simulink model "sm_vehicle_2axle_heave_roll_mu"  (R2025b)
settings: Solver=ode23t  StartTime=0.0  StopTime=14.2  MaxStep=0.2  RelTol=1e-3  AbsTol=1e-3  EnableMultiTasking=on
PostLoadFcn:
  | sm_vehicle_2axle_heave_roll_param
  | sm_vehicle_2axle_heave_roll_scene
  | sm_vehicle_2axle_heave_roll_config_maneuver(bdroot,VehicleData,'plateau');
  | set_param([bdroot '/Vehicle'],'popup_surface_conditions','Checker Right');
StartFcn:
  | tic
StopFcn:
  | Elapsed_Sim_Time = toc;
undefined symbols (not defined in the file): brake_trqTs, Disc, FL, FR, Hydraulic, InitVehicle, Mode, RL, RR, SceneData, valve_maxA, valve_maxO, VehicleData, X, Y, Z
libraries: fl_lib x92, sm_lib x43, nesl_utility x40, sm_vehicle_utilities_lib x21, sdlc_lib x8, SimscapeFluids_lib x8, simulink x2, simulink_extras x1
(part 5 of 5)

== system sm_vehicle_2axle_heave_roll_mu/Brakes/Brakes/Disc/Actuator/Hydraulic/Return Spring FR ==
  Damper : fl_lib/Mechanical/Translational Elements/Translational Damper  D=D N/(m/s)  v_specify=off  v_priority=None  v=0 m/s  v_nominal_specify=off  v_nominal_value=1  v_nominal_unit=m/s  f_specify=off  f_priority=None  f=0 N  f_nominal_specify=off  f_nominal_value=1  f_nominal_unit=N
  Spring : fl_lib/Mechanical/Translational Elements/Translational Spring  spr_rate=spr_rate N/m  v_specify=off  v_priority=None  v=0 m/s  v_nominal_specify=off  v_nominal_value=1  v_nominal_unit=m/s  f_specify=off  f_priority=None  f=0 N  f_nominal_specify=off  f_nominal_value=1  f_nominal_unit=N  x_specify=off  x_priority=High  x=0 m  x_nominal_specify=off  x_nominal_value=1  x_nominal_unit=m
  R : PMIOPort  Side=Right
  C : PMIOPort  Port=2  Side=Left
  connections:
  Damper/LConn1 -- R/RConn1 -- Spring/LConn1
  C/RConn1 -- Damper/RConn1 -- Spring/RConn1

== system sm_vehicle_2axle_heave_roll_mu/Brakes/Brakes/Disc/Actuator/Hydraulic/Return Spring RL ==
  Damper : fl_lib/Mechanical/Translational Elements/Translational Damper  D=D N/(m/s)  v_specify=off  v_priority=None  v=0 m/s  v_nominal_specify=off  v_nominal_value=1  v_nominal_unit=m/s  f_specify=off  f_priority=None  f=0 N  f_nominal_specify=off  f_nominal_value=1  f_nominal_unit=N
  Spring : fl_lib/Mechanical/Translational Elements/Translational Spring  spr_rate=spr_rate N/m  v_specify=off  v_priority=None  v=0 m/s  v_nominal_specify=off  v_nominal_value=1  v_nominal_unit=m/s  f_specify=off  f_priority=None  f=0 N  f_nominal_specify=off  f_nominal_value=1  f_nominal_unit=N  x_specify=off  x_priority=High  x=0 m  x_nominal_specify=off  x_nominal_value=1  x_nominal_unit=m
  R : PMIOPort  Side=Right
  C : PMIOPort  Port=2  Side=Left
  connections:
  R/RConn1 -- Damper/LConn1 -- Spring/LConn1
  C/RConn1 -- Spring/RConn1 -- Damper/RConn1

== system sm_vehicle_2axle_heave_roll_mu/Brakes/Brakes/Disc/Actuator/Hydraulic/Return Spring RR ==
  Damper : fl_lib/Mechanical/Translational Elements/Translational Damper  D=D N/(m/s)  v_specify=off  v_priority=None  v=0 m/s  v_nominal_specify=off  v_nominal_value=1  v_nominal_unit=m/s  f_specify=off  f_priority=None  f=0 N  f_nominal_specify=off  f_nominal_value=1  f_nominal_unit=N
  Spring : fl_lib/Mechanical/Translational Elements/Translational Spring  spr_rate=spr_rate N/m  v_specify=off  v_priority=None  v=0 m/s  v_nominal_specify=off  v_nominal_value=1  v_nominal_unit=m/s  f_specify=off  f_priority=None  f=0 N  f_nominal_specify=off  f_nominal_value=1  f_nominal_unit=N  x_specify=off  x_priority=High  x=0 m  x_nominal_specify=off  x_nominal_value=1  x_nominal_unit=m
  R : PMIOPort  Side=Right
  C : PMIOPort  Port=2  Side=Left
  connections:
  Spring/RConn1 -- Damper/RConn1 -- C/RConn1
  Spring/LConn1 -- R/RConn1 -- Damper/LConn1

== system sm_vehicle_2axle_heave_roll_mu/Brakes/Brakes/Disc/Actuator/Ideal/Actuator Dynamics FL ==
  In : Inport
  Gain : Gain  Gain=1./b
  Integrator : Integrator  InitialCondition=x_initial.*b
  Sum : Sum  Inputs=|+-  InputSameDT=on  SaturateOnIntegerOverflow=on  OutDataTypeStr=Inherit: Same as first input
  Out : Outport  VectorParamsAs1DForOutWhenUnconnected=off
  wires:
  Sum/1 -> Integrator/1
  In/1 -> Sum/1
  Integrator/1 -> Gain/1
  Gain/1 -> Sum/2, Out/1

== system sm_vehicle_2axle_heave_roll_mu/Brakes/Brakes/Disc/Actuator/Ideal/Actuator Dynamics FR ==
  In : Inport
  Gain : Gain  Gain=1./b
  Integrator : Integrator  InitialCondition=x_initial.*b
  Sum : Sum  Inputs=|+-  InputSameDT=on  SaturateOnIntegerOverflow=on  OutDataTypeStr=Inherit: Same as first input
  Out : Outport  VectorParamsAs1DForOutWhenUnconnected=off
  wires:
  Gain/1 -> Out/1, Sum/2
  Integrator/1 -> Gain/1
  In/1 -> Sum/1
  Sum/1 -> Integrator/1

== system sm_vehicle_2axle_heave_roll_mu/Brakes/Brakes/Disc/Actuator/Ideal/Actuator Dynamics RL ==
  In : Inport
  Gain : Gain  Gain=1./b
  Integrator : Integrator  InitialCondition=x_initial.*b
  Sum : Sum  Inputs=|+-  InputSameDT=on  SaturateOnIntegerOverflow=on  OutDataTypeStr=Inherit: Same as first input
  Out : Outport  VectorParamsAs1DForOutWhenUnconnected=off
  wires:
  Gain/1 -> Out/1, Sum/2
  Integrator/1 -> Gain/1
  In/1 -> Sum/1
  Sum/1 -> Integrator/1

== system sm_vehicle_2axle_heave_roll_mu/Brakes/Brakes/Disc/Actuator/Ideal/Actuator Dynamics RR ==
  In : Inport
  Gain : Gain  Gain=1./b
  Integrator : Integrator  InitialCondition=x_initial.*b
  Sum : Sum  Inputs=|+-  InputSameDT=on  SaturateOnIntegerOverflow=on  OutDataTypeStr=Inherit: Same as first input
  Out : Outport  VectorParamsAs1DForOutWhenUnconnected=off
  wires:
  Sum/1 -> Integrator/1
  In/1 -> Sum/1
  Integrator/1 -> Gain/1
  Gain/1 -> Sum/2, Out/1

== system sm_vehicle_2axle_heave_roll_mu/Brakes/Brakes/Disc/Actuator/Ideal/Front Piston Area ==
  Cylinder Bore : Constant  Value=d_caliper_bore_f
  Gain pi div 4 : Gain  Gain=pi/4
  Square : Math  Operator=square  SignedPower=on
  area : Outport  VectorParamsAs1DForOutWhenUnconnected=off
  wires:
  Square/1 -> Gain pi div 4/1
  Cylinder Bore/1 -> Square/1
  Gain pi div 4/1 -> area/1

== system sm_vehicle_2axle_heave_roll_mu/Brakes/Brakes/Disc/Actuator/Ideal/Rear Piston Area ==
  Cylinder Bore : Constant  Value=d_caliper_bore_r
  Gain pi div 4 : Gain  Gain=pi/4
  Square : Math  Operator=square  SignedPower=on
  area : Outport  VectorParamsAs1DForOutWhenUnconnected=off
  wires:
  Gain pi div 4/1 -> area/1
  Cylinder Bore/1 -> Square/1
  Square/1 -> Gain pi div 4/1

== system sm_vehicle_2axle_heave_roll_mu/Brakes/Brakes/Disc/Actuator/Ideal/Return Spring FL ==
  Damper : fl_lib/Mechanical/Translational Elements/Translational Damper  D=D N/(m/s)  v_specify=off  v_priority=None  v=0 m/s  v_nominal_specify=off  v_nominal_value=1  v_nominal_unit=m/s  f_specify=off  f_priority=None  f=0 N  f_nominal_specify=off  f_nominal_value=1  f_nominal_unit=N
  Spring : fl_lib/Mechanical/Translational Elements/Translational Spring  spr_rate=spr_rate N/m  v_specify=off  v_priority=None  v=0 m/s  v_nominal_specify=off  v_nominal_value=1  v_nominal_unit=m/s  f_specify=off  f_priority=None  f=0 N  f_nominal_specify=off  f_nominal_value=1  f_nominal_unit=N  x_specify=off  x_priority=High  x=0 m  x_nominal_specify=off  x_nominal_value=1  x_nominal_unit=m
  R : PMIOPort  Side=Right
  C : PMIOPort  Port=2  Side=Left
  connections:
  Damper/LConn1 -- R/RConn1 -- Spring/LConn1
  C/RConn1 -- Damper/RConn1 -- Spring/RConn1

== system sm_vehicle_2axle_heave_roll_mu/Brakes/Brakes/Disc/Actuator/Ideal/Return Spring FR ==
  Damper : fl_lib/Mechanical/Translational Elements/Translational Damper  D=D N/(m/s)  v_specify=off  v_priority=None  v=0 m/s  v_nominal_specify=off  v_nominal_value=1  v_nominal_unit=m/s  f_specify=off  f_priority=None  f=0 N  f_nominal_specify=off  f_nominal_value=1  f_nominal_unit=N
  Spring : fl_lib/Mechanical/Translational Elements/Translational Spring  spr_rate=spr_rate N/m  v_specify=off  v_priority=None  v=0 m/s  v_nominal_specify=off  v_nominal_value=1  v_nominal_unit=m/s  f_specify=off  f_priority=None  f=0 N  f_nominal_specify=off  f_nominal_value=1  f_nominal_unit=N  x_specify=off  x_priority=High  x=0 m  x_nominal_specify=off  x_nominal_value=1  x_nominal_unit=m
  R : PMIOPort  Side=Right
  C : PMIOPort  Port=2  Side=Left
  connections:
  Spring/RConn1 -- Damper/RConn1 -- C/RConn1
  Spring/LConn1 -- R/RConn1 -- Damper/LConn1

== system sm_vehicle_2axle_heave_roll_mu/Brakes/Brakes/Disc/Actuator/Ideal/Return Spring RL ==
  Damper : fl_lib/Mechanical/Translational Elements/Translational Damper  D=D N/(m/s)  v_specify=off  v_priority=None  v=0 m/s  v_nominal_specify=off  v_nominal_value=1  v_nominal_unit=m/s  f_specify=off  f_priority=None  f=0 N  f_nominal_specify=off  f_nominal_value=1  f_nominal_unit=N
  Spring : fl_lib/Mechanical/Translational Elements/Translational Spring  spr_rate=spr_rate N/m  v_specify=off  v_priority=None  v=0 m/s  v_nominal_specify=off  v_nominal_value=1  v_nominal_unit=m/s  f_specify=off  f_priority=None  f=0 N  f_nominal_specify=off  f_nominal_value=1  f_nominal_unit=N  x_specify=off  x_priority=High  x=0 m  x_nominal_specify=off  x_nominal_value=1  x_nominal_unit=m
  R : PMIOPort  Side=Right
  C : PMIOPort  Port=2  Side=Left
  connections:
  Damper/RConn1 -- Spring/RConn1 -- C/RConn1
  Spring/LConn1 -- Damper/LConn1 -- R/RConn1

== system sm_vehicle_2axle_heave_roll_mu/Brakes/Brakes/Disc/Actuator/Ideal/Return Spring RR ==
  Damper : fl_lib/Mechanical/Translational Elements/Translational Damper  D=D N/(m/s)  v_specify=off  v_priority=None  v=0 m/s  v_nominal_specify=off  v_nominal_value=1  v_nominal_unit=m/s  f_specify=off  f_priority=None  f=0 N  f_nominal_specify=off  f_nominal_value=1  f_nominal_unit=N
  Spring : fl_lib/Mechanical/Translational Elements/Translational Spring  spr_rate=spr_rate N/m  v_specify=off  v_priority=None  v=0 m/s  v_nominal_specify=off  v_nominal_value=1  v_nominal_unit=m/s  f_specify=off  f_priority=None  f=0 N  f_nominal_specify=off  f_nominal_value=1  f_nominal_unit=N  x_specify=off  x_priority=High  x=0 m  x_nominal_specify=off  x_nominal_value=1  x_nominal_unit=m
  R : PMIOPort  Side=Right
  C : PMIOPort  Port=2  Side=Left
  connections:
  Damper/LConn1 -- R/RConn1 -- Spring/LConn1
  C/RConn1 -- Damper/RConn1 -- Spring/RConn1

== system sm_vehicle_2axle_heave_roll_mu/Brakes/Brakes/Disc/Actuator/Valves/Return Spring FL ==
  Damper : fl_lib/Mechanical/Translational Elements/Translational Damper  D=D N/(m/s)  v_specify=off  v_priority=None  v=0 m/s  v_nominal_specify=off  v_nominal_value=1  v_nominal_unit=m/s  f_specify=off  f_priority=None  f=0 N  f_nominal_specify=off  f_nominal_value=1  f_nominal_unit=N
  Spring : fl_lib/Mechanical/Translational Elements/Translational Spring  spr_rate=spr_rate N/m  v_specify=off  v_priority=None  v=0 m/s  v_nominal_specify=off  v_nominal_value=1  v_nominal_unit=m/s  f_specify=off  f_priority=None  f=0 N  f_nominal_specify=off  f_nominal_value=1  f_nominal_unit=N  x_specify=off  x_priority=High  x=0 m  x_nominal_specify=off  x_nominal_value=1  x_nominal_unit=m
  R : PMIOPort  Side=Right
  C : PMIOPort  Port=2  Side=Left
  connections:
  Damper/LConn1 -- R/RConn1 -- Spring/LConn1
  C/RConn1 -- Damper/RConn1 -- Spring/RConn1

== system sm_vehicle_2axle_heave_roll_mu/Brakes/Brakes/Disc/Actuator/Valves/Return Spring FR ==
  Damper : fl_lib/Mechanical/Translational Elements/Translational Damper  D=D N/(m/s)  v_specify=off  v_priority=None  v=0 m/s  v_nominal_specify=off  v_nominal_value=1  v_nominal_unit=m/s  f_specify=off  f_priority=None  f=0 N  f_nominal_specify=off  f_nominal_value=1  f_nominal_unit=N
  Spring : fl_lib/Mechanical/Translational Elements/Translational Spring  spr_rate=spr_rate N/m  v_specify=off  v_priority=None  v=0 m/s  v_nominal_specify=off  v_nominal_value=1  v_nominal_unit=m/s  f_specify=off  f_priority=None  f=0 N  f_nominal_specify=off  f_nominal_value=1  f_nominal_unit=N  x_specify=off  x_priority=High  x=0 m  x_nominal_specify=off  x_nominal_value=1  x_nominal_unit=m
  R : PMIOPort  Side=Right
  C : PMIOPort  Port=2  Side=Left
  connections:
  Spring/RConn1 -- Damper/RConn1 -- C/RConn1
  Spring/LConn1 -- R/RConn1 -- Damper/LConn1

== system sm_vehicle_2axle_heave_roll_mu/Brakes/Brakes/Disc/Actuator/Valves/Return Spring RL ==
  Damper : fl_lib/Mechanical/Translational Elements/Translational Damper  D=D N/(m/s)  v_specify=off  v_priority=None  v=0 m/s  v_nominal_specify=off  v_nominal_value=1  v_nominal_unit=m/s  f_specify=off  f_priority=None  f=0 N  f_nominal_specify=off  f_nominal_value=1  f_nominal_unit=N
  Spring : fl_lib/Mechanical/Translational Elements/Translational Spring  spr_rate=spr_rate N/m  v_specify=off  v_priority=None  v=0 m/s  v_nominal_specify=off  v_nominal_value=1  v_nominal_unit=m/s  f_specify=off  f_priority=None  f=0 N  f_nominal_specify=off  f_nominal_value=1  f_nominal_unit=N  x_specify=off  x_priority=High  x=0 m  x_nominal_specify=off  x_nominal_value=1  x_nominal_unit=m
  R : PMIOPort  Side=Right
  C : PMIOPort  Port=2  Side=Left
  connections:
  Damper/RConn1 -- Spring/RConn1 -- C/RConn1
  Spring/LConn1 -- Damper/LConn1 -- R/RConn1

== system sm_vehicle_2axle_heave_roll_mu/Brakes/Brakes/Disc/Actuator/Valves/Return Spring RR ==
  Damper : fl_lib/Mechanical/Translational Elements/Translational Damper  D=D N/(m/s)  v_specify=off  v_priority=None  v=0 m/s  v_nominal_specify=off  v_nominal_value=1  v_nominal_unit=m/s  f_specify=off  f_priority=None  f=0 N  f_nominal_specify=off  f_nominal_value=1  f_nominal_unit=N
  Spring : fl_lib/Mechanical/Translational Elements/Translational Spring  spr_rate=spr_rate N/m  v_specify=off  v_priority=None  v=0 m/s  v_nominal_specify=off  v_nominal_value=1  v_nominal_unit=m/s  f_specify=off  f_priority=None  f=0 N  f_nominal_specify=off  f_nominal_value=1  f_nominal_unit=N  x_specify=off  x_priority=High  x=0 m  x_nominal_specify=off  x_nominal_value=1  x_nominal_unit=m
  R : PMIOPort  Side=Right
  C : PMIOPort  Port=2  Side=Left
  connections:
  Damper/LConn1 -- R/RConn1 -- Spring/LConn1
  C/RConn1 -- Damper/RConn1 -- Spring/RConn1

== system sm_vehicle_2axle_heave_roll_mu/Brakes/Brakes/Disc/Actuator/Valves/Sensing pFL ==
  Hydraulic Pressure Sensor : fl_lib/Isothermal Liquid/Sensors/Pressure Sensor (IL)  pressure_measure=foundation.enum.pressure_measure.difference
      settings: InternalSimscapePortConfiguration="{\"Bottom\":[],\"Left\":[{\"id\":\"A\",\"label\":\"A\",\"type\":\"foundation.isothermal_liquid.isothermal_liquid\"}],\"Right\":[{\"id\":\"B\",\"label\":\"B\",\"type\":\"foundation.isothermal_liquid.isothermal_liquid\"},{\"id\":\"P\",\"label\":\"P\",\"type\":\"output\"}],\"Top\":[]}"
      settings: LibrarySourceBlock=|
      | fl_lib/Hydraulic/Hydraulic Sensors/Hydraulic Pressure
      | Sensor
  Hydraulic Reference : fl_lib/Isothermal Liquid/Elements/Reservoir (IL)  reservoir_type=foundation.enum.constant_controlled.constant  pressure_spec=foundation.enum.pressure_spec.atmospheric  reservoir_pressure=0.101325 MPa
      settings: LibrarySourceBlock=fl_lib/Hydraulic/Hydraulic Elements/Hydraulic Reference
  PS-Simulink Converter : nesl_utility/PS-Simulink Converter  PhysicalDomain=network_engine_domain  SubClassName=ps_output  LeftPortType=input  RightPortType=output  PseudoPeriodic=off  Frequencies=[]  VectorFormat=1-D array  Unit=psi  AffineConversion=off
  A : PMIOPort  Side=Left
  p : Outport  VectorParamsAs1DForOutWhenUnconnected=off
  wires:
  PS-Simulink Converter/1 -> p/1
  connections:
  Hydraulic Pressure Sensor/RConn2 -- PS-Simulink Converter/LConn1
  Hydraulic Pressure Sensor/LConn1 -- A/RConn1
  Hydraulic Reference/LConn1 -- Hydraulic Pressure Sensor/RConn1

== system sm_vehicle_2axle_heave_roll_mu/Brakes/Brakes/Disc/Actuator/Valves/Sensing pFR ==
  Hydraulic Pressure Sensor : fl_lib/Isothermal Liquid/Sensors/Pressure Sensor (IL)  pressure_measure=foundation.enum.pressure_measure.difference
      settings: InternalSimscapePortConfiguration="{\"Bottom\":[],\"Left\":[{\"id\":\"A\",\"label\":\"A\",\"type\":\"foundation.isothermal_liquid.isothermal_liquid\"}],\"Right\":[{\"id\":\"B\",\"label\":\"B\",\"type\":\"foundation.isothermal_liquid.isothermal_liquid\"},{\"id\":\"P\",\"label\":\"P\",\"type\":\"output\"}],\"Top\":[]}"
      settings: LibrarySourceBlock=|
      | fl_lib/Hydraulic/Hydraulic Sensors/Hydraulic Pressure
      | Sensor
  Hydraulic Reference : fl_lib/Isothermal Liquid/Elements/Reservoir (IL)  reservoir_type=foundation.enum.constant_controlled.constant  pressure_spec=foundation.enum.pressure_spec.atmospheric  reservoir_pressure=0.101325 MPa
      settings: LibrarySourceBlock=fl_lib/Hydraulic/Hydraulic Elements/Hydraulic Reference
  PS-Simulink Converter : nesl_utility/PS-Simulink Converter  PhysicalDomain=network_engine_domain  SubClassName=ps_output  LeftPortType=input  RightPortType=output  PseudoPeriodic=off  Frequencies=[]  VectorFormat=1-D array  Unit=psi  AffineConversion=off
  A : PMIOPort  Side=Left
  p : Outport  VectorParamsAs1DForOutWhenUnconnected=off
  wires:
  PS-Simulink Converter/1 -> p/1
  connections:
  Hydraulic Reference/LConn1 -- Hydraulic Pressure Sensor/RConn1
  Hydraulic Pressure Sensor/LConn1 -- A/RConn1
  Hydraulic Pressure Sensor/RConn2 -- PS-Simulink Converter/LConn1

== system sm_vehicle_2axle_heave_roll_mu/Brakes/Brakes/Disc/Actuator/Valves/Sensing pRL ==
  Hydraulic Pressure Sensor : fl_lib/Isothermal Liquid/Sensors/Pressure Sensor (IL)  pressure_measure=foundation.enum.pressure_measure.difference
      settings: InternalSimscapePortConfiguration="{\"Bottom\":[],\"Left\":[{\"id\":\"A\",\"label\":\"A\",\"type\":\"foundation.isothermal_liquid.isothermal_liquid\"}],\"Right\":[{\"id\":\"B\",\"label\":\"B\",\"type\":\"foundation.isothermal_liquid.isothermal_liquid\"},{\"id\":\"P\",\"label\":\"P\",\"type\":\"output\"}],\"Top\":[]}"
      settings: LibrarySourceBlock=|
      | fl_lib/Hydraulic/Hydraulic Sensors/Hydraulic Pressure
      | Sensor
  Hydraulic Reference : fl_lib/Isothermal Liquid/Elements/Reservoir (IL)  reservoir_type=foundation.enum.constant_controlled.constant  pressure_spec=foundation.enum.pressure_spec.atmospheric  reservoir_pressure=0.101325 MPa
      settings: LibrarySourceBlock=fl_lib/Hydraulic/Hydraulic Elements/Hydraulic Reference
  PS-Simulink Converter : nesl_utility/PS-Simulink Converter  PhysicalDomain=network_engine_domain  SubClassName=ps_output  LeftPortType=input  RightPortType=output  PseudoPeriodic=off  Frequencies=[]  VectorFormat=1-D array  Unit=psi  AffineConversion=off
  A : PMIOPort  Side=Left
  p : Outport  VectorParamsAs1DForOutWhenUnconnected=off
  wires:
  PS-Simulink Converter/1 -> p/1
  connections:
  Hydraulic Reference/LConn1 -- Hydraulic Pressure Sensor/RConn1
  Hydraulic Pressure Sensor/LConn1 -- A/RConn1
  Hydraulic Pressure Sensor/RConn2 -- PS-Simulink Converter/LConn1

== system sm_vehicle_2axle_heave_roll_mu/Brakes/Brakes/Disc/Actuator/Valves/Sensing pRR ==
  Hydraulic Pressure Sensor : fl_lib/Isothermal Liquid/Sensors/Pressure Sensor (IL)  pressure_measure=foundation.enum.pressure_measure.difference
      settings: InternalSimscapePortConfiguration="{\"Bottom\":[],\"Left\":[{\"id\":\"A\",\"label\":\"A\",\"type\":\"foundation.isothermal_liquid.isothermal_liquid\"}],\"Right\":[{\"id\":\"B\",\"label\":\"B\",\"type\":\"foundation.isothermal_liquid.isothermal_liquid\"},{\"id\":\"P\",\"label\":\"P\",\"type\":\"output\"}],\"Top\":[]}"
      settings: LibrarySourceBlock=|
      | fl_lib/Hydraulic/Hydraulic Sensors/Hydraulic Pressure
      | Sensor
  Hydraulic Reference : fl_lib/Isothermal Liquid/Elements/Reservoir (IL)  reservoir_type=foundation.enum.constant_controlled.constant  pressure_spec=foundation.enum.pressure_spec.atmospheric  reservoir_pressure=0.101325 MPa
      settings: LibrarySourceBlock=fl_lib/Hydraulic/Hydraulic Elements/Hydraulic Reference
  PS-Simulink Converter : nesl_utility/PS-Simulink Converter  PhysicalDomain=network_engine_domain  SubClassName=ps_output  LeftPortType=input  RightPortType=output  PseudoPeriodic=off  Frequencies=[]  VectorFormat=1-D array  Unit=psi  AffineConversion=off
  A : PMIOPort  Side=Left
  p : Outport  VectorParamsAs1DForOutWhenUnconnected=off
  wires:
  PS-Simulink Converter/1 -> p/1
  connections:
  Hydraulic Pressure Sensor/RConn2 -- PS-Simulink Converter/LConn1
  Hydraulic Pressure Sensor/LConn1 -- A/RConn1
  Hydraulic Reference/LConn1 -- Hydraulic Pressure Sensor/RConn1

== system sm_vehicle_2axle_heave_roll_mu/Brakes/Brakes/Disc/Actuator/Valves/Valves FL ==
  S : Inport
  Actuator Dynamics : Subsystem  mask(First-order lag supporting vector signals){b=brkTs, x_initial=0}
      mask prompts: b "Filter time constant"; x_initial "Initial output"
      mask help: Models a lag of the form 1/(b*s+1) where s is the Laplace operator.
  Demux : Demux  Outputs=2
  Orifice Apply : SimscapeFluids_lib/Isothermal Liquid/Valves & Orifices/Orifices/Orifice (IL)  orifice_type=foundation.enum.constant_variable.variable  constant_orifice_spec=fluids.isothermal_liquid.valves_orifices.orifices.enum.constant_orifice_spec.area  variable_orifice_spec=1  orifice_area_constant=1e-3 m^2  p_diff_TLU_constant=[-4, -3, -2, -1, -.5, 0, .5, 1, 2, 3, 4] MPa  vol_flow_TLU_constant=[-2.44, -2.12, -1.68, -1.22, -.84, 0, .85, 1.21, 1.7, 2.09, 2.41] .* 1e-3 m^3/s  S_min=(open_max_apply)/(area_max_apply)*(1e-12) - (0) m  del_S=(-(0) + (open_max_apply)) - ((open_max_apply)/(area_max_apply)*(1e-12) - (0)) m  open_orientation=1  area_max=area_max_apply m^2  area_leak=1e-12 m^2  S_TLU=[-.002, 0, .002, .005, .015] - (0) m  orifice_area_TLU=[1e-09, 2.0352e-07, 4.0736e-05, .00011438, .00034356] m^2  area=inf m^2  Cd=0.7  Re_c=150  smoothing_factor=0  pressure_recovery=false  S_vol_flow_TLU=[-.002, 0, .002, .005, .015] - (0) m  p_diff_TLU=[-10000000, -5000000, -2000000, 2000000, 5000000, 10000000] Pa  vol_flow_TLU=[-1e-07, -7.0711e-08, -4.4721e-08, 4.4721e-08, 7.0711e-08, 1e-07; -2.0352e-05, -1.4391e-05, -9.1017e-06, 9.1017e-06, 1.4391e-05, 2.0352e-05; -.0040736, -.0028805, -.0018218, .0018218, .0028805, .0040736; -.011438, -.0080879, -.0051152, .0051152, .0080879, .011438; -.034356, -.024293, -.015364, .015364, .024293, .034356] m^3/s
      settings: LibrarySourceBlock=sh_lib/Orifices/Variable Orifice  InternalSimscapePortConfiguration="{\"Bottom\":[],\"Left\":[{\"id\":\"A\",\"label\":\"A\",\"type\":\"foundation.isothermal_liquid.isothermal_liquid\"},{\"id\":\"S\",\"label\":\"S\",\"type\":\"input\"}],\"Right\":[{\"id\":\"B\",\"label\":\"B\",\"type\":\"foundation.isothermal_liquid.isothermal_liquid\"}],\"Top\":[]}"
  Orifice Release : SimscapeFluids_lib/Isothermal Liquid/Valves & Orifices/Orifices/Orifice (IL)  orifice_type=foundation.enum.constant_variable.variable  constant_orifice_spec=fluids.isothermal_liquid.valves_orifices.orifices.enum.constant_orifice_spec.area  variable_orifice_spec=1  orifice_area_constant=1e-3 m^2  p_diff_TLU_constant=[-4, -3, -2, -1, -.5, 0, .5, 1, 2, 3, 4] MPa  vol_flow_TLU_constant=[-2.44, -2.12, -1.68, -1.22, -.84, 0, .85, 1.21, 1.7, 2.09, 2.41] .* 1e-3 m^3/s  S_min=(open_max_rel)/(area_max_rel)*(1e-12) - (0) m  del_S=(-(0) + (open_max_rel)) - ((open_max_rel)/(area_max_rel)*(1e-12) - (0)) m  open_orientation=1  area_max=area_max_rel m^2  area_leak=1e-12 m^2  S_TLU=[-.002, 0, .002, .005, .015] - (0) m  orifice_area_TLU=[1e-09, 2.0352e-07, 4.0736e-05, .00011438, .00034356] m^2  area=inf m^2  Cd=0.7  Re_c=150  smoothing_factor=0  pressure_recovery=false  S_vol_flow_TLU=[-.002, 0, .002, .005, .015] - (0) m  p_diff_TLU=[-10000000, -5000000, -2000000, 2000000, 5000000, 10000000] Pa  vol_flow_TLU=[-1e-07, -7.0711e-08, -4.4721e-08, 4.4721e-08, 7.0711e-08, 1e-07; -2.0352e-05, -1.4391e-05, -9.1017e-06, 9.1017e-06, 1.4391e-05, 2.0352e-05; -.0040736, -.0028805, -.0018218, .0018218, .0028805, .0040736; -.011438, -.0080879, -.0051152, .0051152, .0080879, .011438; -.034356, -.024293, -.015364, .015364, .024293, .034356] m^3/s
      settings: LibrarySourceBlock=sh_lib/Orifices/Variable Orifice  InternalSimscapePortConfiguration="{\"Bottom\":[],\"Left\":[{\"id\":\"A\",\"label\":\"A\",\"type\":\"foundation.isothermal_liquid.isothermal_liquid\"},{\"id\":\"S\",\"label\":\"S\",\"type\":\"input\"}],\"Right\":[{\"id\":\"B\",\"label\":\"B\",\"type\":\"foundation.isothermal_liquid.isothermal_liquid\"}],\"Top\":[]}"
  PS Gain : fl_lib/Physical Signals/Functions/PS Gain  gain=open_max_rel
  PS Gain1 : fl_lib/Physical Signals/Functions/PS Gain  gain=open_max_apply
  Simulink-PS Converter : nesl_utility/Simulink-PS Converter  PhysicalDomain=network_engine_domain  SubClassName=ps_input  LeftPortType=input  RightPortType=output  PseudoPeriodic=off  Frequencies=[]  NoiseDistribution=none  NoiseParameters=[]  Unit=1  AffineConversion=off  FilteringAndDerivatives=provide  SimscapeFilterOrder=1  InputFilterTimeConstant=0.001  UdotUserProvided=0
  Simulink-PS Converter1 : nesl_utility/Simulink-PS Converter  PhysicalDomain=network_engine_domain  SubClassName=ps_input  LeftPortType=input  RightPortType=output  PseudoPeriodic=off  Frequencies=[]  NoiseDistribution=none  NoiseParameters=[]  Unit=1  AffineConversion=off  FilteringAndDerivatives=provide  SimscapeFilterOrder=1  InputFilterTimeConstant=0.001  UdotUserProvided=0
  A : PMIOPort  Side=Left
  R : PMIOPort  Port=2  Side=Left
  P : PMIOPort  Port=3  Side=Right
  wires:
  S/1 -> Actuator Dynamics/1(In)
  Demux/1 -> Simulink-PS Converter/1
  Demux/2 -> Simulink-PS Converter1/1
  Actuator Dynamics/1(Out) -> Demux/1
  connections:
  Simulink-PS Converter/RConn1 -- PS Gain/LConn1
  Simulink-PS Converter1/RConn1 -- PS Gain1/LConn1
  Orifice Apply/LConn2 -- PS Gain1/RConn1
  Orifice Apply/LConn1 -- A/RConn1
  Orifice Apply/RConn1 -- Orifice Release/LConn1 -- P/RConn1
  Orifice Release/LConn2 -- PS Gain/RConn1
  Orifice Release/RConn1 -- R/RConn1

== system sm_vehicle_2axle_heave_roll_mu/Brakes/Brakes/Disc/Actuator/Valves/Valves FR ==
  S : Inport
  Actuator Dynamics : Subsystem  mask(First-order lag supporting vector signals){b=brkTs, x_initial=0}
      mask prompts: b "Filter time constant"; x_initial "Initial output"
      mask help: Models a lag of the form 1/(b*s+1) where s is the Laplace operator.
  Demux1 : Demux  Outputs=2
  Orifice Apply : SimscapeFluids_lib/Isothermal Liquid/Valves & Orifices/Orifices/Orifice (IL)  orifice_type=foundation.enum.constant_variable.variable  constant_orifice_spec=fluids.isothermal_liquid.valves_orifices.orifices.enum.constant_orifice_spec.area  variable_orifice_spec=1  orifice_area_constant=1e-3 m^2  p_diff_TLU_constant=[-4, -3, -2, -1, -.5, 0, .5, 1, 2, 3, 4] MPa  vol_flow_TLU_constant=[-2.44, -2.12, -1.68, -1.22, -.84, 0, .85, 1.21, 1.7, 2.09, 2.41] .* 1e-3 m^3/s  S_min=(open_max_apply)/(area_max_apply)*(1e-12) - (0) m  del_S=(-(0) + (open_max_apply)) - ((open_max_apply)/(area_max_apply)*(1e-12) - (0)) m  open_orientation=1  area_max=area_max_apply m^2  area_leak=1e-12 m^2  S_TLU=[-.002, 0, .002, .005, .015] - (0) m  orifice_area_TLU=[1e-09, 2.0352e-07, 4.0736e-05, .00011438, .00034356] m^2  area=inf m^2  Cd=0.7  Re_c=150  smoothing_factor=0  pressure_recovery=false  S_vol_flow_TLU=[-.002, 0, .002, .005, .015] - (0) m  p_diff_TLU=[-10000000, -5000000, -2000000, 2000000, 5000000, 10000000] Pa  vol_flow_TLU=[-1e-07, -7.0711e-08, -4.4721e-08, 4.4721e-08, 7.0711e-08, 1e-07; -2.0352e-05, -1.4391e-05, -9.1017e-06, 9.1017e-06, 1.4391e-05, 2.0352e-05; -.0040736, -.0028805, -.0018218, .0018218, .0028805, .0040736; -.011438, -.0080879, -.0051152, .0051152, .0080879, .011438; -.034356, -.024293, -.015364, .015364, .024293, .034356] m^3/s
      settings: LibrarySourceBlock=sh_lib/Orifices/Variable Orifice  InternalSimscapePortConfiguration="{\"Bottom\":[],\"Left\":[{\"id\":\"A\",\"label\":\"A\",\"type\":\"foundation.isothermal_liquid.isothermal_liquid\"},{\"id\":\"S\",\"label\":\"S\",\"type\":\"input\"}],\"Right\":[{\"id\":\"B\",\"label\":\"B\",\"type\":\"foundation.isothermal_liquid.isothermal_liquid\"}],\"Top\":[]}"
  Orifice Release : SimscapeFluids_lib/Isothermal Liquid/Valves & Orifices/Orifices/Orifice (IL)  orifice_type=foundation.enum.constant_variable.variable  constant_orifice_spec=fluids.isothermal_liquid.valves_orifices.orifices.enum.constant_orifice_spec.area  variable_orifice_spec=1  orifice_area_constant=1e-3 m^2  p_diff_TLU_constant=[-4, -3, -2, -1, -.5, 0, .5, 1, 2, 3, 4] MPa  vol_flow_TLU_constant=[-2.44, -2.12, -1.68, -1.22, -.84, 0, .85, 1.21, 1.7, 2.09, 2.41] .* 1e-3 m^3/s  S_min=(open_max_rel)/(area_max_rel)*(1e-12) - (0) m  del_S=(-(0) + (open_max_rel)) - ((open_max_rel)/(area_max_rel)*(1e-12) - (0)) m  open_orientation=1  area_max=area_max_rel m^2  area_leak=1e-12 m^2  S_TLU=[-.002, 0, .002, .005, .015] - (0) m  orifice_area_TLU=[1e-09, 2.0352e-07, 4.0736e-05, .00011438, .00034356] m^2  area=inf m^2  Cd=0.7  Re_c=150  smoothing_factor=0  pressure_recovery=false  S_vol_flow_TLU=[-.002, 0, .002, .005, .015] - (0) m  p_diff_TLU=[-10000000, -5000000, -2000000, 2000000, 5000000, 10000000] Pa  vol_flow_TLU=[-1e-07, -7.0711e-08, -4.4721e-08, 4.4721e-08, 7.0711e-08, 1e-07; -2.0352e-05, -1.4391e-05, -9.1017e-06, 9.1017e-06, 1.4391e-05, 2.0352e-05; -.0040736, -.0028805, -.0018218, .0018218, .0028805, .0040736; -.011438, -.0080879, -.0051152, .0051152, .0080879, .011438; -.034356, -.024293, -.015364, .015364, .024293, .034356] m^3/s
      settings: LibrarySourceBlock=sh_lib/Orifices/Variable Orifice  InternalSimscapePortConfiguration="{\"Bottom\":[],\"Left\":[{\"id\":\"A\",\"label\":\"A\",\"type\":\"foundation.isothermal_liquid.isothermal_liquid\"},{\"id\":\"S\",\"label\":\"S\",\"type\":\"input\"}],\"Right\":[{\"id\":\"B\",\"label\":\"B\",\"type\":\"foundation.isothermal_liquid.isothermal_liquid\"}],\"Top\":[]}"
  PS Gain : fl_lib/Physical Signals/Functions/PS Gain  gain=open_max_rel
  PS Gain1 : fl_lib/Physical Signals/Functions/PS Gain  gain=open_max_apply
  Simulink-PS Converter2 : nesl_utility/Simulink-PS Converter  PhysicalDomain=network_engine_domain  SubClassName=ps_input  LeftPortType=input  RightPortType=output  PseudoPeriodic=off  Frequencies=[]  NoiseDistribution=none  NoiseParameters=[]  Unit=1  AffineConversion=off  FilteringAndDerivatives=provide  SimscapeFilterOrder=1  InputFilterTimeConstant=0.001  UdotUserProvided=0
  Simulink-PS Converter3 : nesl_utility/Simulink-PS Converter  PhysicalDomain=network_engine_domain  SubClassName=ps_input  LeftPortType=input  RightPortType=output  PseudoPeriodic=off  Frequencies=[]  NoiseDistribution=none  NoiseParameters=[]  Unit=1  AffineConversion=off  FilteringAndDerivatives=provide  SimscapeFilterOrder=1  InputFilterTimeConstant=0.001  UdotUserProvided=0
  A : PMIOPort  Side=Left
  R : PMIOPort  Port=2  Side=Left
  P : PMIOPort  Port=3  Side=Right
  wires:
  S/1 -> Actuator Dynamics/1(In)
  Demux1/2 -> Simulink-PS Converter3/1
  Demux1/1 -> Simulink-PS Converter2/1
  Actuator Dynamics/1(Out) -> Demux1/1
  connections:
  Simulink-PS Converter3/RConn1 -- PS Gain1/LConn1
  Simulink-PS Converter2/RConn1 -- PS Gain/LConn1
  P/RConn1 -- Orifice Release/LConn1 -- Orifice Apply/RConn1
  Orifice Apply/LConn2 -- PS Gain1/RConn1
  Orifice Apply/LConn1 -- A/RConn1
  Orifice Release/LConn2 -- PS Gain/RConn1
  Orifice Release/RConn1 -- R/RConn1

== system sm_vehicle_2axle_heave_roll_mu/Brakes/Brakes/Disc/Actuator/Valves/Valves RL ==
  S : Inport
  Actuator Dynamics : Subsystem  mask(First-order lag supporting vector signals){b=brkTs, x_initial=0}
      mask prompts: b "Filter time constant"; x_initial "Initial output"
      mask help: Models a lag of the form 1/(b*s+1) where s is the Laplace operator.
  Demux3 : Demux  Outputs=2
  Orifice Apply : SimscapeFluids_lib/Isothermal Liquid/Valves & Orifices/Orifices/Orifice (IL)  orifice_type=foundation.enum.constant_variable.variable  constant_orifice_spec=fluids.isothermal_liquid.valves_orifices.orifices.enum.constant_orifice_spec.area  variable_orifice_spec=1  orifice_area_constant=1e-3 m^2  p_diff_TLU_constant=[-4, -3, -2, -1, -.5, 0, .5, 1, 2, 3, 4] MPa  vol_flow_TLU_constant=[-2.44, -2.12, -1.68, -1.22, -.84, 0, .85, 1.21, 1.7, 2.09, 2.41] .* 1e-3 m^3/s  S_min=(open_max_apply)/(area_max_apply)*(1e-12) - (0) m  del_S=(-(0) + (open_max_apply)) - ((open_max_apply)/(area_max_apply)*(1e-12) - (0)) m  open_orientation=1  area_max=area_max_apply m^2  area_leak=1e-12 m^2  S_TLU=[-.002, 0, .002, .005, .015] - (0) m  orifice_area_TLU=[1e-09, 2.0352e-07, 4.0736e-05, .00011438, .00034356] m^2  area=inf m^2  Cd=0.7  Re_c=150  smoothing_factor=0  pressure_recovery=false  S_vol_flow_TLU=[-.002, 0, .002, .005, .015] - (0) m  p_diff_TLU=[-10000000, -5000000, -2000000, 2000000, 5000000, 10000000] Pa  vol_flow_TLU=[-1e-07, -7.0711e-08, -4.4721e-08, 4.4721e-08, 7.0711e-08, 1e-07; -2.0352e-05, -1.4391e-05, -9.1017e-06, 9.1017e-06, 1.4391e-05, 2.0352e-05; -.0040736, -.0028805, -.0018218, .0018218, .0028805, .0040736; -.011438, -.0080879, -.0051152, .0051152, .0080879, .011438; -.034356, -.024293, -.015364, .015364, .024293, .034356] m^3/s
      settings: LibrarySourceBlock=sh_lib/Orifices/Variable Orifice  InternalSimscapePortConfiguration="{\"Bottom\":[],\"Left\":[{\"id\":\"A\",\"label\":\"A\",\"type\":\"foundation.isothermal_liquid.isothermal_liquid\"},{\"id\":\"S\",\"label\":\"S\",\"type\":\"input\"}],\"Right\":[{\"id\":\"B\",\"label\":\"B\",\"type\":\"foundation.isothermal_liquid.isothermal_liquid\"}],\"Top\":[]}"
  Orifice Release : SimscapeFluids_lib/Isothermal Liquid/Valves & Orifices/Orifices/Orifice (IL)  orifice_type=foundation.enum.constant_variable.variable  constant_orifice_spec=fluids.isothermal_liquid.valves_orifices.orifices.enum.constant_orifice_spec.area  variable_orifice_spec=1  orifice_area_constant=1e-3 m^2  p_diff_TLU_constant=[-4, -3, -2, -1, -.5, 0, .5, 1, 2, 3, 4] MPa  vol_flow_TLU_constant=[-2.44, -2.12, -1.68, -1.22, -.84, 0, .85, 1.21, 1.7, 2.09, 2.41] .* 1e-3 m^3/s  S_min=(open_max_rel)/(area_max_rel)*(1e-12) - (0) m  del_S=(-(0) + (open_max_rel)) - ((open_max_rel)/(area_max_rel)*(1e-12) - (0)) m  open_orientation=1  area_max=area_max_rel m^2  area_leak=1e-12 m^2  S_TLU=[-.002, 0, .002, .005, .015] - (0) m  orifice_area_TLU=[1e-09, 2.0352e-07, 4.0736e-05, .00011438, .00034356] m^2  area=inf m^2  Cd=0.7  Re_c=150  smoothing_factor=0  pressure_recovery=false  S_vol_flow_TLU=[-.002, 0, .002, .005, .015] - (0) m  p_diff_TLU=[-10000000, -5000000, -2000000, 2000000, 5000000, 10000000] Pa  vol_flow_TLU=[-1e-07, -7.0711e-08, -4.4721e-08, 4.4721e-08, 7.0711e-08, 1e-07; -2.0352e-05, -1.4391e-05, -9.1017e-06, 9.1017e-06, 1.4391e-05, 2.0352e-05; -.0040736, -.0028805, -.0018218, .0018218, .0028805, .0040736; -.011438, -.0080879, -.0051152, .0051152, .0080879, .011438; -.034356, -.024293, -.015364, .015364, .024293, .034356] m^3/s
      settings: LibrarySourceBlock=sh_lib/Orifices/Variable Orifice  InternalSimscapePortConfiguration="{\"Bottom\":[],\"Left\":[{\"id\":\"A\",\"label\":\"A\",\"type\":\"foundation.isothermal_liquid.isothermal_liquid\"},{\"id\":\"S\",\"label\":\"S\",\"type\":\"input\"}],\"Right\":[{\"id\":\"B\",\"label\":\"B\",\"type\":\"foundation.isothermal_liquid.isothermal_liquid\"}],\"Top\":[]}"
  PS Gain : fl_lib/Physical Signals/Functions/PS Gain  gain=open_max_rel
  PS Gain1 : fl_lib/Physical Signals/Functions/PS Gain  gain=open_max_apply
  Simulink-PS Converter6 : nesl_utility/Simulink-PS Converter  PhysicalDomain=network_engine_domain  SubClassName=ps_input  LeftPortType=input  RightPortType=output  PseudoPeriodic=off  Frequencies=[]  NoiseDistribution=none  NoiseParameters=[]  Unit=1  AffineConversion=off  FilteringAndDerivatives=provide  SimscapeFilterOrder=1  InputFilterTimeConstant=0.001  UdotUserProvided=0
  Simulink-PS Converter7 : nesl_utility/Simulink-PS Converter  PhysicalDomain=network_engine_domain  SubClassName=ps_input  LeftPortType=input  RightPortType=output  PseudoPeriodic=off  Frequencies=[]  NoiseDistribution=none  NoiseParameters=[]  Unit=1  AffineConversion=off  FilteringAndDerivatives=provide  SimscapeFilterOrder=1  InputFilterTimeConstant=0.001  UdotUserProvided=0
  A : PMIOPort  Side=Left
  R : PMIOPort  Port=2  Side=Left
  P : PMIOPort  Port=3  Side=Right
  wires:
  Actuator Dynamics/1(Out) -> Demux3/1
  Demux3/1 -> Simulink-PS Converter6/1
  Demux3/2 -> Simulink-PS Converter7/1
  S/1 -> Actuator Dynamics/1(In)
  connections:
  Simulink-PS Converter7/RConn1 -- PS Gain1/LConn1
  Simulink-PS Converter6/RConn1 -- PS Gain/LConn1
  Orifice Apply/LConn2 -- PS Gain1/RConn1
  Orifice Apply/LConn1 -- A/RConn1
  P/RConn1 -- Orifice Apply/RConn1 -- Orifice Release/LConn1
  Orifice Release/LConn2 -- PS Gain/RConn1
  Orifice Release/RConn1 -- R/RConn1

== system sm_vehicle_2axle_heave_roll_mu/Brakes/Brakes/Disc/Actuator/Valves/Valves RR ==
  S : Inport
  Actuator Dynamics RR : Subsystem  mask(First-order lag supporting vector signals){b=brkTs, x_initial=0}
      mask prompts: b "Filter time constant"; x_initial "Initial output"
      mask help: Models a lag of the form 1/(b*s+1) where s is the Laplace operator.
  Demux2 : Demux  Outputs=2
  Orifice Apply : SimscapeFluids_lib/Isothermal Liquid/Valves & Orifices/Orifices/Orifice (IL)  orifice_type=foundation.enum.constant_variable.variable  constant_orifice_spec=fluids.isothermal_liquid.valves_orifices.orifices.enum.constant_orifice_spec.area  variable_orifice_spec=1  orifice_area_constant=1e-3 m^2  p_diff_TLU_constant=[-4, -3, -2, -1, -.5, 0, .5, 1, 2, 3, 4] MPa  vol_flow_TLU_constant=[-2.44, -2.12, -1.68, -1.22, -.84, 0, .85, 1.21, 1.7, 2.09, 2.41] .* 1e-3 m^3/s  S_min=(open_max_apply)/(area_max_apply)*(1e-12) - (0) m  del_S=(-(0) + (open_max_apply)) - ((open_max_apply)/(area_max_apply)*(1e-12) - (0)) m  open_orientation=1  area_max=area_max_apply m^2  area_leak=1e-12 m^2  S_TLU=[-.002, 0, .002, .005, .015] - (0) m  orifice_area_TLU=[1e-09, 2.0352e-07, 4.0736e-05, .00011438, .00034356] m^2  area=inf m^2  Cd=0.7  Re_c=150  smoothing_factor=0  pressure_recovery=false  S_vol_flow_TLU=[-.002, 0, .002, .005, .015] - (0) m  p_diff_TLU=[-10000000, -5000000, -2000000, 2000000, 5000000, 10000000] Pa  vol_flow_TLU=[-1e-07, -7.0711e-08, -4.4721e-08, 4.4721e-08, 7.0711e-08, 1e-07; -2.0352e-05, -1.4391e-05, -9.1017e-06, 9.1017e-06, 1.4391e-05, 2.0352e-05; -.0040736, -.0028805, -.0018218, .0018218, .0028805, .0040736; -.011438, -.0080879, -.0051152, .0051152, .0080879, .011438; -.034356, -.024293, -.015364, .015364, .024293, .034356] m^3/s
      settings: LibrarySourceBlock=sh_lib/Orifices/Variable Orifice  InternalSimscapePortConfiguration="{\"Bottom\":[],\"Left\":[{\"id\":\"A\",\"label\":\"A\",\"type\":\"foundation.isothermal_liquid.isothermal_liquid\"},{\"id\":\"S\",\"label\":\"S\",\"type\":\"input\"}],\"Right\":[{\"id\":\"B\",\"label\":\"B\",\"type\":\"foundation.isothermal_liquid.isothermal_liquid\"}],\"Top\":[]}"
  Orifice Release : SimscapeFluids_lib/Isothermal Liquid/Valves & Orifices/Orifices/Orifice (IL)  orifice_type=foundation.enum.constant_variable.variable  constant_orifice_spec=fluids.isothermal_liquid.valves_orifices.orifices.enum.constant_orifice_spec.area  variable_orifice_spec=1  orifice_area_constant=1e-3 m^2  p_diff_TLU_constant=[-4, -3, -2, -1, -.5, 0, .5, 1, 2, 3, 4] MPa  vol_flow_TLU_constant=[-2.44, -2.12, -1.68, -1.22, -.84, 0, .85, 1.21, 1.7, 2.09, 2.41] .* 1e-3 m^3/s  S_min=(open_max_rel)/(area_max_rel)*(1e-12) - (0) m  del_S=(-(0) + (open_max_rel)) - ((open_max_rel)/(area_max_rel)*(1e-12) - (0)) m  open_orientation=1  area_max=area_max_rel m^2  area_leak=1e-12 m^2  S_TLU=[-.002, 0, .002, .005, .015] - (0) m  orifice_area_TLU=[1e-09, 2.0352e-07, 4.0736e-05, .00011438, .00034356] m^2  area=inf m^2  Cd=0.7  Re_c=150  smoothing_factor=0  pressure_recovery=false  S_vol_flow_TLU=[-.002, 0, .002, .005, .015] - (0) m  p_diff_TLU=[-10000000, -5000000, -2000000, 2000000, 5000000, 10000000] Pa  vol_flow_TLU=[-1e-07, -7.0711e-08, -4.4721e-08, 4.4721e-08, 7.0711e-08, 1e-07; -2.0352e-05, -1.4391e-05, -9.1017e-06, 9.1017e-06, 1.4391e-05, 2.0352e-05; -.0040736, -.0028805, -.0018218, .0018218, .0028805, .0040736; -.011438, -.0080879, -.0051152, .0051152, .0080879, .011438; -.034356, -.024293, -.015364, .015364, .024293, .034356] m^3/s
      settings: LibrarySourceBlock=sh_lib/Orifices/Variable Orifice  InternalSimscapePortConfiguration="{\"Bottom\":[],\"Left\":[{\"id\":\"A\",\"label\":\"A\",\"type\":\"foundation.isothermal_liquid.isothermal_liquid\"},{\"id\":\"S\",\"label\":\"S\",\"type\":\"input\"}],\"Right\":[{\"id\":\"B\",\"label\":\"B\",\"type\":\"foundation.isothermal_liquid.isothermal_liquid\"}],\"Top\":[]}"
  PS Gain : fl_lib/Physical Signals/Functions/PS Gain  gain=open_max_rel
  PS Gain1 : fl_lib/Physical Signals/Functions/PS Gain  gain=open_max_apply
  Simulink-PS Converter4 : nesl_utility/Simulink-PS Converter  PhysicalDomain=network_engine_domain  SubClassName=ps_input  LeftPortType=input  RightPortType=output  PseudoPeriodic=off  Frequencies=[]  NoiseDistribution=none  NoiseParameters=[]  Unit=1  AffineConversion=off  FilteringAndDerivatives=provide  SimscapeFilterOrder=1  InputFilterTimeConstant=0.001  UdotUserProvided=0
  Simulink-PS Converter5 : nesl_utility/Simulink-PS Converter  PhysicalDomain=network_engine_domain  SubClassName=ps_input  LeftPortType=input  RightPortType=output  PseudoPeriodic=off  Frequencies=[]  NoiseDistribution=none  NoiseParameters=[]  Unit=1  AffineConversion=off  FilteringAndDerivatives=provide  SimscapeFilterOrder=1  InputFilterTimeConstant=0.001  UdotUserProvided=0
  A : PMIOPort  Side=Left
  R : PMIOPort  Port=2  Side=Left
  P : PMIOPort  Port=3  Side=Right
  wires:
  Demux2/1 -> Simulink-PS Converter4/1
  Actuator Dynamics RR/1(Out) -> Demux2/1
  Demux2/2 -> Simulink-PS Converter5/1
  S/1 -> Actuator Dynamics RR/1(In)
  connections:
  Simulink-PS Converter4/RConn1 -- PS Gain/LConn1
  PS Gain1/LConn1 -- Simulink-PS Converter5/RConn1
  Orifice Apply/LConn2 -- PS Gain1/RConn1
  Orifice Apply/LConn1 -- A/RConn1
  Orifice Apply/RConn1 -- Orifice Release/LConn1 -- P/RConn1
  Orifice Release/LConn2 -- PS Gain/RConn1
  Orifice Release/RConn1 -- R/RConn1

== system sm_vehicle_2axle_heave_roll_mu/Brakes/Brakes/Disc/Actuator/Valves/Valves FL/Actuator Dynamics ==
  In : Inport
  Gain : Gain  Gain=1./b
  Integrator : Integrator  InitialCondition=x_initial.*b
  Sum : Sum  Inputs=|+-  InputSameDT=on  SaturateOnIntegerOverflow=on  OutDataTypeStr=Inherit: Same as first input
  Out : Outport  VectorParamsAs1DForOutWhenUnconnected=off
  wires:
  Sum/1 -> Integrator/1
  In/1 -> Sum/1
  Integrator/1 -> Gain/1
  Gain/1 -> Sum/2, Out/1

== system sm_vehicle_2axle_heave_roll_mu/Brakes/Brakes/Disc/Actuator/Valves/Valves FR/Actuator Dynamics ==
  In : Inport
  Gain : Gain  Gain=1./b
  Integrator : Integrator  InitialCondition=x_initial.*b
  Sum : Sum  Inputs=|+-  InputSameDT=on  SaturateOnIntegerOverflow=on  OutDataTypeStr=Inherit: Same as first input
  Out : Outport  VectorParamsAs1DForOutWhenUnconnected=off
  wires:
  Gain/1 -> Out/1, Sum/2
  Integrator/1 -> Gain/1
  In/1 -> Sum/1
  Sum/1 -> Integrator/1

== system sm_vehicle_2axle_heave_roll_mu/Brakes/Brakes/Disc/Actuator/Valves/Valves RL/Actuator Dynamics ==
  In : Inport
  Gain : Gain  Gain=1./b
  Integrator : Integrator  InitialCondition=x_initial.*b
  Sum : Sum  Inputs=|+-  InputSameDT=on  SaturateOnIntegerOverflow=on  OutDataTypeStr=Inherit: Same as first input
  Out : Outport  VectorParamsAs1DForOutWhenUnconnected=off
  wires:
  Gain/1 -> Out/1, Sum/2
  Integrator/1 -> Gain/1
  In/1 -> Sum/1
  Sum/1 -> Integrator/1

== system sm_vehicle_2axle_heave_roll_mu/Brakes/Brakes/Disc/Actuator/Valves/Valves RR/Actuator Dynamics RR ==
  In : Inport
  Gain : Gain  Gain=1./b
  Integrator : Integrator  InitialCondition=x_initial.*b
  Sum : Sum  Inputs=|+-  InputSameDT=on  SaturateOnIntegerOverflow=on  OutDataTypeStr=Inherit: Same as first input
  Out : Outport  VectorParamsAs1DForOutWhenUnconnected=off
  wires:
  Sum/1 -> Integrator/1
  In/1 -> Sum/1
  Integrator/1 -> Gain/1
  Gain/1 -> Sum/2, Out/1
